simulink model "simulink_sample_model"  (R2017a)
settings: Solver=VariableStepAuto  StartTime=0.0  StopTime=40.0  RelTol=1e-6
settings Model: Creator=mrc.classroom  LastModifiedBy=mrc.classroom

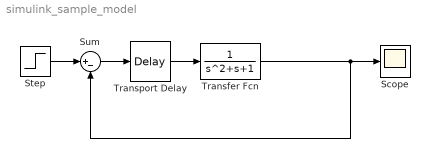
== system simulink_sample_model ==
  Scope : Scope
  Step : Step  SampleTime=0
  Sum : Sum  Inputs=|+-
  Transfer Fcn : TransferFcn  Denominator=[1 1 1]
  Transport Delay : TransportDelay  DelayTime=2.3
  wires:
  Transfer Fcn/1 -> Sum/2, Scope/1
  Step/1 -> Sum/1
  Sum/1 -> Transport Delay/1
  Transport Delay/1 -> Transfer Fcn/1
